simulink model "electricalSystem"  (R2021a)
settings: Solver=VariableStepAuto  StartTime=0.0  StopTime=4  RelTol=1e-3
model workspace (MAT data in the model file):
  C = 1e-06
  L = 0.001
  R = 1
  Vdc = 30
libraries: spsSeriesRLCBranchLib x2, spsCurrentMeasurementLib x1, spsDCVoltageSourceLib x1, spsMosfetLib x1, spsVoltageMeasurementLib x1, spspowerguiLib x1
settings Model: Creator=User  LastModifiedBy=User

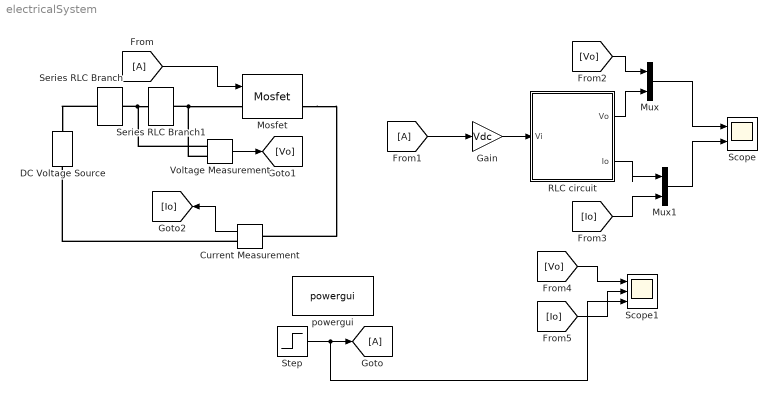
== system electricalSystem ==
  Current Measurement : spsCurrentMeasurementLib/Current Measurement  PhasorSimulation=off  OutputType=Complex  PSBequivalent=0
  DC Voltage Source : spsDCVoltageSourceLib/DC Voltage Source  Amplitude=Vdc  Measurements=None
  Gain : Gain  Gain=Vdc
  Mosfet : spsMosfetLib/Mosfet  Ron=0.1  Lon=0  Rd=0.01  Vfd=0  IC=0  Rs=1e5  Cs=inf  Measurements=on
  Mux : Mux  Inputs=2
  Mux1 : Mux  Inputs=2
  RLC circuit : Subsystem
  Scope : Scope  NumInputPorts=2
  Scope1 : Scope  NumInputPorts=3
  Series RLC Branch : spsSeriesRLCBranchLib/Series RLC Branch  LConnTagsString=__new0  RConnTagsString=__new0  BranchType=R  Resistance=R  Inductance=1e-3  SetiL0=off  InitialCurrent=0  Capacitance=1e-6  Setx0=off  InitialVoltage=0  Measurements=None
  Series RLC Branch1 : spsSeriesRLCBranchLib/Series RLC Branch  LConnTagsString=__new0  RConnTagsString=__new0  BranchType=C  Resistance=R  Inductance=1e-3  SetiL0=off  InitialCurrent=0  Capacitance=C  Setx0=on  InitialVoltage=0  Measurements=None
  Step : Step  SampleTime=0
  Voltage Measurement : spsVoltageMeasurementLib/Voltage Measurement  PhasorSimulation=off  OutputType=Complex  PSBequivalent=0
  powergui : spspowerguiLib/powergui  Priority=1  SimulationMode=Continuous  SampleTime=50e-6  frequency=60  Iterations=50  frequencyindice=0  Pbase=100e6  ErrMax=1e-4  UnitsV=kV  UnitsW=MW  buscounter=0  FunctionMessages=off  echomessages=off  EnableUseOfTLC=off  CurrentSourceSwitches=off  DisableSnubberDevices=off  DisableRonSwitches=off  DisableVfSwitches=off  DisplayEquations=off  AutomaticDiscreteSolvers=off  SolverType=Tustin/Backward Euler (TBE)  Interpol=off  ExternalGateDelay=off  methode=off  Ts=100  x0status=blocks  SPID=on  SwTol=0  HookPort=off  NonlinearTolerance=1e-4  nMaxIteration=100  ContinueOnMaxIteration=off  RestoreLinks=warning  ResistiveCurrentMeasurement=off  Frange=[0:2:500]  Ylog=off  Xlog=on  ShowGrid=off  save=off  variable=ZData  structure=0  ZoomFFT=off  StartTime=0.0  cycles=1  DisplayStyle=1  fundamental=60  FreqAxis=off  MaxFrequency=1000  frequencyindicesteady=1  RmsSteady=1  display=off
  wires:
  Gain/1 -> RLC circuit/1(Vi)
  Step/1 -> Scope1/3, [A]
  [A] -> Mosfet/1
  [A] -> Gain/1
  Voltage Measurement/1 -> [Vo]
  [Vo] -> Mux/1
  RLC circuit/1(Vo) -> Mux/2
  Mux/1 -> Scope/1
  RLC circuit/2(Io) -> Mux1/1
  Mux1/1 -> Scope/2
  Current Measurement/1 -> [Io]
  [Io] -> Mux1/2
  [Vo] -> Scope1/1
  [Io] -> Scope1/2
  connections:
  Series RLC Branch1/RConn1 -- Voltage Measurement/LConn2 -- Mosfet/LConn1
  Series RLC Branch/LConn1 -- DC Voltage Source/RConn1
  Mosfet/RConn1 -- Current Measurement/LConn1
  Voltage Measurement/LConn1 -- Series RLC Branch1/LConn1 -- Series RLC Branch/RConn1
  Current Measurement/RConn1 -- DC Voltage Source/LConn1

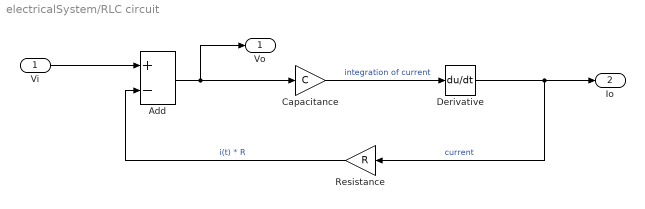
== system electricalSystem/RLC circuit ==
  Vi : Inport
  Add : Sum  Inputs=+-
  Capacitance : Gain  Gain=C
  Derivative : Derivative
  Resistance : Gain  Gain=R
  Vo : Outport
  Io : Outport  Port=2
  wires:
  Derivative/1 -> Io/1, Resistance/1  "current"
  Add/1 -> Vo/1, Capacitance/1
  Vi/1 -> Add/1
  Resistance/1 -> Add/2  "i(t) * R"
  Capacitance/1 -> Derivative/1  "integration of current"
